simulink model "check"  (R2019a)
settings: Solver=VariableStepAuto  StartTime=0.0  StopTime=10  RelTol=1e-3
libraries: shared6dof x1
settings Model: Creator=rob  LastModifiedBy=rob

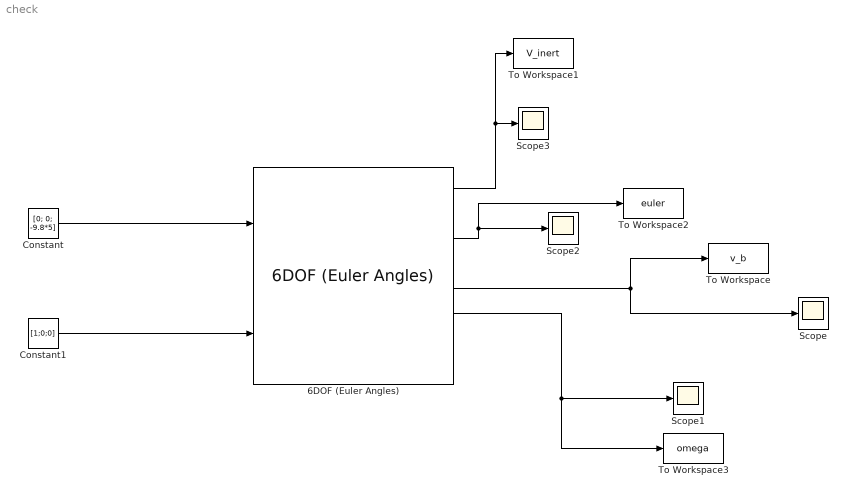
== system check ==
  6DOF (Euler Angles) : shared6dof/6DOF (Euler Angles)  units=Metric (MKS)  mtype=Fixed  rep=Euler Angles  xme_0=[0 0 0]  Vm_0=[0 0 0]  eul_0=[0 0 0]  pm_0=[1 0 0]  mass_0=5.0  mass_e=0.5  mass_f=2.0  inertia=I  inertia_e=eye(3)  inertia_f=2*eye(3)  k_quat=1.0  vre_flag=on  abi_flag=off  aMode=0  xme_statename=''  Vm_statename=''  eul_statename=''  quat_statename=''  pm_statename=''  mass_statename=''
      settings: SourceProductBaseCode=AE
  Constant : Constant  Value=[0; 0; -9.8*5]
  Constant1 : Constant  Value=[1;0;0]
  Scope{,1..3} (4 alike) : Scope
  To Workspace : ToWorkspace  VariableName=v_b  SaveFormat=Timeseries  SampleTime=-1
  To Workspace1 : ToWorkspace  VariableName=V_inert  SaveFormat=Timeseries  SampleTime=-1
  To Workspace2 : ToWorkspace  VariableName=euler  SaveFormat=Timeseries  SampleTime=-1
  To Workspace3 : ToWorkspace  VariableName=omega  SaveFormat=Timeseries  SampleTime=-1
  wires:
  Constant/1 -> 6DOF (Euler Angles)/1
  Constant1/1 -> 6DOF (Euler Angles)/2
  6DOF (Euler Angles)/5 -> Scope/1, To Workspace/1
  6DOF (Euler Angles)/6 -> To Workspace3/1, Scope1/1
  6DOF (Euler Angles)/3 -> To Workspace2/1, Scope2/1
  6DOF (Euler Angles)/1 -> To Workspace1/1, Scope3/1
